simulink library "FF_Library"  (R2024b)
settings: Solver=VariableStepAuto  StartTime=0.0  StopTime=10.0  RelTol=1e-3
undefined symbols (not defined in the file or in its folder): Slope1, Slope2
libraries: simulink x60
(part 2 of 4)

== system FF_Library/Counter&Timer/CounterCycle_SourceZero ==
  Chart : Stateflow chart  TreatAsAtomicUnit=on
  Ts1 : Constant  Value=CounterCycle  OutDataTypeStr=Inherit: Inherit via back propagation  SampleTime=-1
      settings: AttributesFormatString=%<value>
      mask Display:
      | try
      | set_param(gcb,'AttributesFormatString','%<value>');% get the value name
      | % Constant=get_param(gcb,'Value');
      | % set_param(gcb,'Name',Constant,'ShowName','on');
      | end
      | try
      | Constant=get_param(gcb,'Value');
      | Constant_value=[Constant '.Value'];
      | Constant_type=[Constant '.DataType'];
      | Constant_value= evalin('base',Constant_value);% get the data name
      | Constant_type=evalin('base',Constant_type);% get the data type
      |           if strcmp(Constant_type,'boolean')||strcmp(Constant_type,'xpDT_Bool')% If the datatype is boolean
      |             if size(Constant_value)==[1 1]
      |                   if Constant_value==1
      |                     disp('True');
      |                   else
      |                     disp('False');
      |                   end
      |             else
      |                 disp(Constant_value);
      |             end
      |           else
      |              try
      |                  if mod(Constant_value,1)==0 &&(strcmp(Constant_type,'single')||strcmp(Constant_type,'xpDT_Single'))
      |                  fprintf('%.1f',Constant_value); %Display at least 1 decimal if DataType is 'single'
      |                  else
      |                  disp(Constant_value);
      |                  end
      |              catch
      |              disp(Constant_value);
      |              end
      |            end
      | catch
      |     try
      |        Constant_value= evalin('base',Constant);
      |        disp(num2str(Constant_value));
      |     catch
      |       color('blue');
      |       disp('NoData');
      |    end
      | end
      | %%  Created By Gmh 2018.06.28  %%
      | %%  Modified By Gmh 2018.10.24  %%
  Ts2 : Constant  Value=0  OutDataTypeStr=Inherit: Inherit via back propagation  SampleTime=-1
      settings: AttributesFormatString=%<value>
      mask Display:
      | try
      | set_param(gcb,'AttributesFormatString','%<value>');% get the value name
      | % Constant=get_param(gcb,'Value');
      | % set_param(gcb,'Name',Constant,'ShowName','on');
      | end
      | try
      | Constant=get_param(gcb,'Value');
      | Constant_value=[Constant '.Value'];
      | Constant_type=[Constant '.DataType'];
      | Constant_value= evalin('base',Constant_value);% get the data name
      | Constant_type=evalin('base',Constant_type);% get the data type
      |           if strcmp(Constant_type,'boolean')||strcmp(Constant_type,'xpDT_Bool')% If the datatype is boolean
      |             if size(Constant_value)==[1 1]
      |                   if Constant_value==1
      |                     disp('True');
      |                   else
      |                     disp('False');
      |                   end
      |             else
      |                 disp(Constant_value);
      |             end
      |           else
      |              try
      |                  if mod(Constant_value,1)==0 &&(strcmp(Constant_type,'single')||strcmp(Constant_type,'xpDT_Single'))
      |                  fprintf('%.1f',Constant_value); %Display at least 1 decimal if DataType is 'single'
      |                  else
      |                  disp(Constant_value);
      |                  end
      |              catch
      |              disp(Constant_value);
      |              end
      |            end
      | catch
      |     try
      |        Constant_value= evalin('base',Constant);
      |        disp(num2str(Constant_value));
      |     catch
      |       color('blue');
      |       disp('NoData');
      |    end
      | end
      | %%  Created By Gmh 2018.06.28  %%
      | %%  Modified By Gmh 2018.10.24  %%
  Ts3 : Constant  OutDataTypeStr=Inherit: Inherit via back propagation  SampleTime=-1
      settings: AttributesFormatString=%<value>
      mask Display:
      | try
      | set_param(gcb,'AttributesFormatString','%<value>');% get the value name
      | % Constant=get_param(gcb,'Value');
      | % set_param(gcb,'Name',Constant,'ShowName','on');
      | end
      | try
      | Constant=get_param(gcb,'Value');
      | Constant_value=[Constant '.Value'];
      | Constant_type=[Constant '.DataType'];
      | Constant_value= evalin('base',Constant_value);% get the data name
      | Constant_type=evalin('base',Constant_type);% get the data type
      |           if strcmp(Constant_type,'boolean')||strcmp(Constant_type,'xpDT_Bool')% If the datatype is boolean
      |             if size(Constant_value)==[1 1]
      |                   if Constant_value==1
      |                     disp('True');
      |                   else
      |                     disp('False');
      |                   end
      |             else
      |                 disp(Constant_value);
      |             end
      |           else
      |              try
      |                  if mod(Constant_value,1)==0 &&(strcmp(Constant_type,'single')||strcmp(Constant_type,'xpDT_Single'))
      |                  fprintf('%.1f',Constant_value); %Display at least 1 decimal if DataType is 'single'
      |                  else
      |                  disp(Constant_value);
      |                  end
      |              catch
      |              disp(Constant_value);
      |              end
      |            end
      | catch
      |     try
      |        Constant_value= evalin('base',Constant);
      |        disp(num2str(Constant_value));
      |     catch
      |       color('blue');
      |       disp('NoData');
      |    end
      | end
      | %%  Created By Gmh 2018.06.28  %%
      | %%  Modified By Gmh 2018.10.24  %%
  Cnt : Outport  VectorParamsAs1DForOutWhenUnconnected=off
  wires:
  Ts1/1 -> Chart/3(CounterCycle)
  Ts3/1 -> Chart/1(Enable)
  Ts2/1 -> Chart/2(InitValue)
  Chart/1(Cnt) -> Cnt/1

== system FF_Library/Counter&Timer/TIMER_RE ==
  note: y
  note: x1_out
  dT : Inport
  E : Inport  Port=2
  R : Inport  Port=3
  IV : Inport  Port=4
  x_in : Inport  Port=5
  Functionality : Subsystem
  y : Outport
  x_out : Outport  Port=2
  wires:
  dT/1 -> Functionality/4(dT)
  R/1 -> Functionality/2(R)
  Functionality/2(x_out) -> x_out/1
  IV/1 -> Functionality/3(IV)
  x_in/1 -> Functionality/5(x_in)
  Functionality/1(y) -> y/1
  E/1 -> Functionality/1(E)

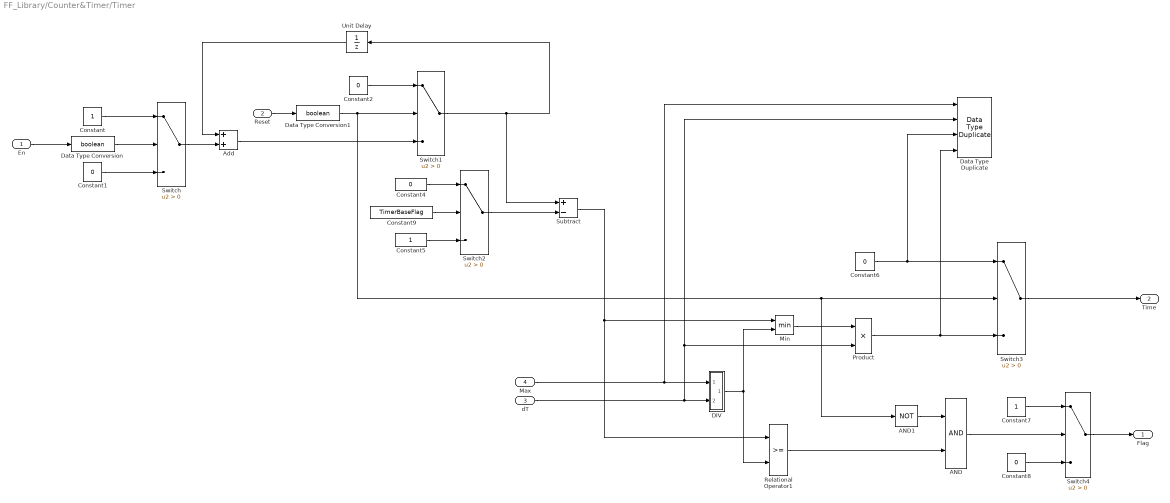
== system FF_Library/Counter&Timer/Timer ==
  En : Inport
  Reset : Inport  Port=2
  dT : Inport  Port=3
  Max : Inport  Port=4
  AND : Logic  AllPortsSameDT=off  OutDataTypeStr=boolean
  AND1 : Logic  Operator=NOT  AllPortsSameDT=off  OutDataTypeStr=boolean
  Add : Sum  OutDataTypeStr=single  SaturateOnIntegerOverflow=on
  Constant : Constant  OutDataTypeStr=boolean
  Constant{1..2,4,8} (4 alike) : Constant  Value=0  OutDataTypeStr=boolean
  Constant5 : Constant  OutDataTypeStr=boolean
  Constant6 : Constant  Value=0  OutDataTypeStr=Inherit: Inherit via back propagation
  Constant7 : Constant  OutDataTypeStr=boolean
  Constant9 : Constant  Value=TimerBaseFlag  OutDataTypeStr=boolean
  DIV : Subsystem  mask(DIV){MinRange=1e-15}
      mask prompts: MinRange "smallest allowed value to divide by"
      mask help:
      | 除法模块：
      | 带有除0保护。
      mask Display:
      | port_label('input',1,'×');
      | port_label('input',2,'÷');
      | port_label('output',1,'');
  Data Type Duplicate : DataTypeDuplicate  NumInputPorts=4
  Data Type Conversion : DataTypeConversion  OutDataTypeStr=boolean  RndMeth=Floor
  Data Type Conversion1 : DataTypeConversion  OutDataTypeStr=boolean  RndMeth=Floor
  Min : MinMax  Inputs=2
  Product : Product  OutDataTypeStr=Inherit: Inherit via back propagation  SaturateOnIntegerOverflow=on
  Relational Operator1 : RelationalOperator  OutDataTypeStr=boolean  RndMeth=Simplest  InputSameDT=off
  Subtract : Sum  Inputs=+-  SaturateOnIntegerOverflow=on
  Switch{,1..3} (4 alike) : Switch  Criteria=u2 > Threshold  InputSameDT=off
  Switch4 : Switch  Criteria=u2 > Threshold  OutDataTypeStr=boolean  InputSameDT=off
  Unit Delay : UnitDelay  InputProcessing=Columns as channels (frame based)  SampleTime=-1  HasFrameUpgradeWarning=on
  Flag : Outport
  Time : Outport  Port=2
  wires:
  Unit Delay/1 -> Add/1
  Constant9/1 -> Switch2/2
  Subtract/1 -> Relational Operator1/1, Min/1
  Add/1 -> Switch1/3
  Constant4/1 -> Switch2/1
  Switch3/1 -> Time/1
  DIV/1(Out1) -> Relational Operator1/2, Min/2
  Data Type Conversion1/1 -> Switch1/2, Switch3/2, AND1/1
  Constant2/1 -> Switch1/1
  Constant8/1 -> Switch4/3
  Constant6/1 -> Switch3/1, Data Type Duplicate/3
  Constant5/1 -> Switch2/3
  Constant/1 -> Switch/1
  AND1/1 -> AND/1
  Switch2/1 -> Subtract/2
  AND/1 -> Switch4/2
  Constant1/1 -> Switch/3
  Min/1 -> Product/1
  Constant7/1 -> Switch4/1
  Product/1 -> Switch3/3, Data Type Duplicate/4
  dT/1 -> Data Type Duplicate/2, Product/2, DIV/2(In2)
  Reset/1 -> Data Type Conversion1/1
  Switch1/1 -> Unit Delay/1, Subtract/1
  Switch/1 -> Add/2
  Data Type Conversion/1 -> Switch/2
  En/1 -> Data Type Conversion/1
  Switch4/1 -> Flag/1
  Max/1 -> Data Type Duplicate/1, DIV/1(In1)
  Relational Operator1/1 -> AND/2

== system FF_Library/Ctrl/INTEGRATORK_REL ==
  note: x_out
  note: B_max
  note: B_min
  note: y
  MX : Inport
  MN : Inport  Port=2
  K : Inport  Port=3
  dT : Inport  Port=4
  u : Inport  Port=5
  E : Inport  Port=6
  R : Inport  Port=7
  IV : Inport  Port=8
  x_in : Inport  Port=9
  Functionality : Subsystem
  y : Terminator
  B_min : Outport
  B_max : Outport  Port=2
  x_out : Outport  Port=3
  wires:
  Functionality/2(B_min) -> B_min/1
  Functionality/1(y) -> y/1
  u/1 -> Functionality/5(u)
  MX/1 -> Functionality/1(MX)
  E/1 -> Functionality/6(E)
  R/1 -> Functionality/7(R)
  MN/1 -> Functionality/2(MN)
  Functionality/3(B_max) -> B_max/1
  Functionality/4(x_out) -> x_out/1
  IV/1 -> Functionality/8(IV)
  K/1 -> Functionality/3(K)
  dT/1 -> Functionality/4(dT)
  x_in/1 -> Functionality/9(x_in)

== system FF_Library/Ctrl/INTEGRATORT_REL ==
  note: x_out
  note: B_max
  note: B_min
  note: y
  MX : Inport
  MN : Inport  Port=2
  T : Inport  Port=3
  dT : Inport  Port=4
  u : Inport  Port=5
  E : Inport  Port=6
  R : Inport  Port=7
  IV : Inport  Port=8
  x_in : Inport  Port=9
  Functionality : Subsystem
  y : Terminator
  B_min : Outport
  B_max : Outport  Port=2
  x_out : Outport  Port=3
  wires:
  Functionality/2(B_min) -> B_min/1
  Functionality/1(y) -> y/1
  u/1 -> Functionality/5(u)
  MX/1 -> Functionality/1(MX)
  E/1 -> Functionality/6(E)
  R/1 -> Functionality/7(R)
  MN/1 -> Functionality/2(MN)
  Functionality/3(B_max) -> B_max/1
  Functionality/4(x_out) -> x_out/1
  IV/1 -> Functionality/8(IV)
  T/1 -> Functionality/3(T)
  dT/1 -> Functionality/4(dT)
  x_in/1 -> Functionality/9(x_in)

== system FF_Library/Ctrl/Integrator ==
  Ini : Inport  OutDataTypeStr=boolean
  X : Inport  Port=2  OutDataTypeStr=single
  dT : Inport  Port=3  OutDataTypeStr=single
  Add1 : Sum
  Add2 : Sum
  Constant1 : Constant  Value=0  OutDataTypeStr=single
  Constant3 : Constant  Value=0  OutDataTypeStr=single
  Constant4 : Constant  Value=0.5  OutDataTypeStr=single
  Delay : Delay  DelayLength=1
  Delay1 : Delay  DelayLength=1
  Product : Product  Inputs=3
  Switch : Switch  Criteria=u2 > Threshold  OutDataTypeStr=single  SaturateOnIntegerOverflow=off  InputSameDT=off
  Switch1 : Switch  Criteria=u2 > Threshold  OutDataTypeStr=single  SaturateOnIntegerOverflow=off  InputSameDT=off
  Switch2 : Switch  Criteria=u2 > Threshold  OutDataTypeStr=single  SaturateOnIntegerOverflow=off  InputSameDT=off
  Y : Outport
  wires:
  dT/1 -> Product/1
  Delay/1 -> Switch1/3
  X/1 -> Delay/1, Switch/3
  Constant1/1 -> Switch2/1
  Constant3/1 -> Switch1/1, Switch/1
  Constant4/1 -> Product/2
  Add1/1 -> Y/1, Delay1/1
  Product/1 -> Add1/1
  Switch1/1 -> Add2/2
  Switch/1 -> Add2/1
  Add2/1 -> Product/3
  Delay1/1 -> Switch2/3
  Switch2/1 -> Add1/2
  Ini/1 -> Switch2/2, Switch1/2, Switch/2

== system FF_Library/Ctrl/PID ==
  err : Inport
  E : Inport  Port=2
  DefaultValue : Inport  Port=3
  FeedForward : Inport  Port=4
  Kp : Inport  Port=5
  Kd : Inport  Port=6
  Ki : Inport  Port=7
  Deadband : Inport  Port=8
  Ki_IV : Inport  Port=9
  UpperLimit : Inport  Port=10
  LowerLimit : Inport  Port=11
  Data Type Duplicate1 : DataTypeDuplicate  NumInputPorts=10
  PID : Subsystem
  PID_out : Outport
  wires:
  err/1 -> PID/1(err), Data Type Duplicate1/10
  Ki/1 -> PID/7(Ki), Data Type Duplicate1/5
  Deadband/1 -> PID/9(Deadband), Data Type Duplicate1/3
  Kp/1 -> PID/5(Kp), Data Type Duplicate1/7
  Kd/1 -> PID/6(Kd), Data Type Duplicate1/6
  FeedForward/1 -> PID/4(FeedForward), Data Type Duplicate1/8
  Ki_IV/1 -> PID/8(Ki_IV), Data Type Duplicate1/4
  PID/1(PID_out) -> PID_out/1
  E/1 -> PID/2(E)
  DefaultValue/1 -> PID/3(DefaultValue), Data Type Duplicate1/9
  LowerLimit/1 -> Data Type Duplicate1/1, PID/11(LowerLimit)
  UpperLimit/1 -> PID/10(UpperLimit), Data Type Duplicate1/2

== system FF_Library/Ctrl/PID_Norm ==
  Err : Inport
  Kp : Inport  Port=2
  Ki : Inport  Port=3
  Kd : Inport  Port=4
  Add : Sum  Inputs=+++  RndMeth=Nearest  SaturateOnIntegerOverflow=on
  Product : Product  RndMeth=Nearest  SaturateOnIntegerOverflow=on  OutDataTypeStr=Inherit: Same as first input
  Product1 : Product  RndMeth=Nearest  SaturateOnIntegerOverflow=on  OutDataTypeStr=Inherit: Same as first input
  Product2 : Product  RndMeth=Nearest  SaturateOnIntegerOverflow=on  OutDataTypeStr=Inherit: Same as first input
  Subtract : Sum  Inputs=+-  RndMeth=Nearest  SaturateOnIntegerOverflow=on  OutDataTypeStr=Inherit: Same as first input
  Subtract1 : Sum  RndMeth=Nearest  SaturateOnIntegerOverflow=on  OutDataTypeStr=Inherit: Same as first input
  Unit Delay : UnitDelay  SampleTime=-1  HasFrameUpgradeWarning=on
  Unit Delay1 : UnitDelay  SampleTime=-1  HasFrameUpgradeWarning=on
  PID_out : Outport
  wires:
  Product/1 -> Add/1
  Kp/1 -> Product/1
  Err/1 -> Subtract/1, Product2/1, Unit Delay/1, Product/2
  Subtract/1 -> Product1/1
  Product1/1 -> Add/2
  Ki/1 -> Product2/2
  Unit Delay/1 -> Subtract/2
  Product2/1 -> Subtract1/1
  Add/1 -> PID_out/1
  Kd/1 -> Product1/2
  Subtract1/1 -> Unit Delay1/1, Add/3
  Unit Delay1/1 -> Subtract1/2

== system FF_Library/Delay/TURNOFFDELAYSAMPLE ==
  note: x_out
  note: y
  n : Inport
  u : Inport  Port=2
  R : Inport  Port=3
  x_in : Inport  Port=4
  Functionality : Subsystem
  Rounding Function : Rounding  Operator=round
  y : Outport
  x_out : Outport  Port=2
  wires:
  x_in/1 -> Functionality/4(x_in)
  Functionality/2(x_out) -> x_out/1
  Functionality/1(y) -> y/1
  u/1 -> Functionality/2(u)
  n/1 -> Rounding Function/1
  R/1 -> Functionality/3(R)
  Rounding Function/1 -> Functionality/1(n)

== system FF_Library/Delay/TURNONDELAYSAMPLE ==
  note: x_out
  note: y
  R : Inport
  u : Inport  Port=2
  n : Inport  Port=3
  x_in : Inport  Port=4
  Functionality : Subsystem
  Rounding Function : Rounding  Operator=round
  y : Outport
  x_out : Outport  Port=2
  wires:
  x_in/1 -> Functionality/4(x_in)
  n/1 -> Rounding Function/1
  u/1 -> Functionality/2(u)
  R/1 -> Functionality/3(R)
  Functionality/2(x_out) -> x_out/1
  Functionality/1(y) -> y/1
  Rounding Function/1 -> Functionality/1(n)

== system FF_Library/Delay/TurnOffDeb ==
  u : Inport
  dT : Inport  Port=2
  T : Inport  Port=3
  AND : Logic  AllPortsSameDT=off  OutDataTypeStr=boolean
  AND1 : Logic  Operator=OR  AllPortsSameDT=off  OutDataTypeStr=boolean
  Constant : Constant  Value=0  OutDataTypeStr=Inherit: Inherit via back propagation
  Constant1 : Constant  Value=2  OutDataTypeStr=Inherit: Inherit via back propagation
  Constant2 : Constant  Value=0  OutDataTypeStr=Inherit: Inherit via back propagation
  DIV1 : Subsystem  mask(DIV){MinRange=1e-15}
      mask prompts: MinRange "smallest allowed value to divide by"
      mask help:
      | 除法模块：
      | 带有除0保护。
      mask Display:
      | port_label('input',1,'×');
      | port_label('input',2,'÷');
      | port_label('output',1,'');
  Data Type Duplicate : DataTypeDuplicate  NumInputPorts=4
  Max : MinMax  Function=max  Inputs=2
  NOT : Logic  Operator=NOT  AllPortsSameDT=off  OutDataTypeStr=boolean
  Relational Operator : RelationalOperator  Operator=>  OutDataTypeStr=boolean  RndMeth=Simplest  InputSameDT=off
  Subtract : Sum  Inputs=+-  SaturateOnIntegerOverflow=on
  Subtract2 : Sum  Inputs=+-  SaturateOnIntegerOverflow=on
  Switch : Switch  Criteria=u2 > Threshold  RndMeth=Nearest  InputSameDT=off
  Unit Delay : UnitDelay  SampleTime=-1  HasFrameUpgradeWarning=on
  Unit Delay1 : UnitDelay  SampleTime=-1  HasFrameUpgradeWarning=on
  y : Outport
  wires:
  u/1 -> Unit Delay/1, AND1/1, NOT/1
  NOT/1 -> AND/1
  Unit Delay/1 -> AND/2
  Relational Operator/1 -> AND1/2
  Constant/1 -> Relational Operator/2
  Switch/1 -> Data Type Duplicate/1, Unit Delay1/1, Relational Operator/1
  AND/1 -> Switch/2
  dT/1 -> DIV1/1(In1), Subtract/2, Data Type Duplicate/3
  Constant1/1 -> DIV1/2(In2), Data Type Duplicate/2
  T/1 -> Subtract2/1, Data Type Duplicate/4
  DIV1/1(Out1) -> Subtract2/2
  Unit Delay1/1 -> Subtract/1
  Constant2/1 -> Max/2
  Subtract/1 -> Max/1
  Max/1 -> Switch/3
  AND1/1 -> y/1
  Subtract2/1 -> Switch/1

== system FF_Library/Delay/TurnOffDelay ==
  X : Inport
  Delay : Inport  Port=2
  dT : Inport  Port=3
  Ini : Inport  Port=4
  ADD_blk1 : Sum  InputSameDT=on  OutDataTypeStr=Inherit: Same as first input
      settings: AttributesFormatString=Same input type: %<InputSameDT>
  AND : Logic  AllPortsSameDT=off  OutDataTypeStr=boolean
  CNST_FALSE : Constant  Value=0  OutDataTypeStr=boolean
  CNST_TRUE : Constant  OutDataTypeStr=boolean
  CNST_ZERO : Constant  Value=0  OutDataTypeStr=Inherit: Inherit via back propagation
  DLY_timer : UnitDelay  SampleTime=-1  HasFrameUpgradeWarning=on
      settings: AttributesFormatString=|
      | init = %<InitialCondition>
      | tsample = %<SampleTime>
  Delay1 : Delay  DelayLength=1  InputProcessing=Columns as channels (frame based)
  NOT1 : Logic  Operator=NOT  AllPortsSameDT=off  OutDataTypeStr=boolean
  OR : Logic  Operator=OR  AllPortsSameDT=off  OutDataTypeStr=boolean
  OR_blk : Logic  Operator=OR  OutDataTypeStr=boolean
  REL_blk : RelationalOperator  Operator=>  OutDataTypeStr=boolean  RndMeth=Simplest
  SWT_state : Switch  Criteria=u2 ~= 0  SaturateOnIntegerOverflow=off
      settings: AttributesFormatString=|
      | %<Criteria>
      | Same input type: %<InputSameDT>
  SWT_timer : Switch  Criteria=u2 ~= 0  SaturateOnIntegerOverflow=off
      settings: AttributesFormatString=|
      | %<Criteria>
      | Same input type: %<InputSameDT>
  Y : Outport  VectorParamsAs1DForOutWhenUnconnected=off
  wires:
  SWT_timer/1 -> REL_blk/1, DLY_timer/1
  Delay/1 -> REL_blk/2
  Ini/1 -> OR_blk/2
  X/1 -> OR/1, OR_blk/1
  DLY_timer/1 -> ADD_blk1/2
  OR_blk/1 -> SWT_timer/2
  ADD_blk1/1 -> SWT_timer/3
  dT/1 -> ADD_blk1/1
  CNST_ZERO/1 -> SWT_timer/1
  SWT_state/1 -> Delay1/1, Y/1
  CNST_FALSE/1 -> SWT_state/3
  CNST_TRUE/1 -> SWT_state/1
  REL_blk/1 -> NOT1/1
  OR/1 -> SWT_state/2
  AND/1 -> OR/2
  NOT1/1 -> AND/1
  Delay1/1 -> AND/2

== system FF_Library/Delay/TurnOnDeb ==
  u : Inport
  dT : Inport  Port=2
  T : Inport  Port=3
  AND : Logic  AllPortsSameDT=off  OutDataTypeStr=boolean
  AND1 : Logic  AllPortsSameDT=off  OutDataTypeStr=boolean
  Constant : Constant  Value=0  OutDataTypeStr=Inherit: Inherit via back propagation
  Constant1 : Constant  Value=2  OutDataTypeStr=Inherit: Inherit via back propagation
  Constant2 : Constant  Value=0  OutDataTypeStr=Inherit: Inherit via back propagation
  DIV : Subsystem  mask(DIV){MinRange=1e-15}
      mask prompts: MinRange "smallest allowed value to divide by"
      mask help:
      | 除法模块：
      | 带有除0保护。
      mask Display:
      | port_label('input',1,'×');
      | port_label('input',2,'÷');
      | port_label('output',1,'');
  Data Type Duplicate : DataTypeDuplicate  NumInputPorts=4
  Max : MinMax  Function=max  Inputs=2
  NOT1 : Logic  Operator=NOT  AllPortsSameDT=off  OutDataTypeStr=boolean
  Relational Operator : RelationalOperator  Operator=<=  OutDataTypeStr=boolean  RndMeth=Simplest  InputSameDT=off
  Subtract : Sum  Inputs=+-  SaturateOnIntegerOverflow=on
  Subtract1 : Sum  Inputs=+-  SaturateOnIntegerOverflow=on
  Switch : Switch  Criteria=u2 > Threshold  InputSameDT=off
  Unit Delay : UnitDelay  SampleTime=-1  HasFrameUpgradeWarning=on
  Unit Delay1 : UnitDelay  SampleTime=-1  HasFrameUpgradeWarning=on
  y : Outport
  wires:
  Constant2/1 -> Max/2
  Unit Delay1/1 -> Subtract1/1
  dT/1 -> DIV/1(In1), Subtract1/2, Data Type Duplicate/3
  Subtract1/1 -> Max/1
  AND1/1 -> y/1
  Switch/1 -> Data Type Duplicate/1, Unit Delay1/1, Relational Operator/1
  Unit Delay/1 -> NOT1/1
  T/1 -> Subtract/1, Data Type Duplicate/4
  Relational Operator/1 -> AND1/2
  DIV/1(Out1) -> Subtract/2
  AND/1 -> Switch/2
  Constant/1 -> Relational Operator/2
  u/1 -> AND/1, AND1/1, Unit Delay/1
  Max/1 -> Switch/3
  Constant1/1 -> DIV/2(In2), Data Type Duplicate/2
  Subtract/1 -> Switch/1
  NOT1/1 -> AND/2

== system FF_Library/Delay/TurnOnDelay ==
  X : Inport
  Delay : Inport  Port=2
  dT : Inport  Port=3
  Ini : Inport  Port=4
  ADD_blk1 : Sum  InputSameDT=on  OutDataTypeStr=Inherit: Same as first input
      settings: AttributesFormatString=Same input type: %<InputSameDT>
  CNST_FALSE : Constant  Value=0  OutDataTypeStr=boolean
  CNST_TRUE : Constant  OutDataTypeStr=boolean
  CNST_ZERO : Constant  Value=0  OutDataTypeStr=Inherit: Inherit via back propagation
  DLY_timer : UnitDelay  SampleTime=-1  HasFrameUpgradeWarning=on
      settings: AttributesFormatString=|
      | init = %<InitialCondition>
      | tsample = %<SampleTime>
  NOT_blk3 : Logic  Operator=NOT  OutDataTypeStr=boolean
  OR_blk : Logic  Operator=OR  OutDataTypeStr=boolean
  REL_blk : RelationalOperator  Operator=>  OutDataTypeStr=boolean  RndMeth=Simplest
  SWT_state : Switch  Criteria=u2 ~= 0  SaturateOnIntegerOverflow=off
      settings: AttributesFormatString=|
      | %<Criteria>
      | Same input type: %<InputSameDT>
  SWT_timer : Switch  Criteria=u2 ~= 0  SaturateOnIntegerOverflow=off
      settings: AttributesFormatString=|
      | %<Criteria>
      | Same input type: %<InputSameDT>
  Y : Outport  VectorParamsAs1DForOutWhenUnconnected=off
  wires:
  SWT_timer/1 -> REL_blk/1, DLY_timer/1
  Delay/1 -> REL_blk/2
  OR_blk/1 -> SWT_timer/2
  Ini/1 -> OR_blk/2
  NOT_blk3/1 -> OR_blk/1
  DLY_timer/1 -> ADD_blk1/2
  CNST_FALSE/1 -> SWT_state/3
  X/1 -> NOT_blk3/1
  ADD_blk1/1 -> SWT_timer/3
  CNST_TRUE/1 -> SWT_state/1
  dT/1 -> ADD_blk1/1
  CNST_ZERO/1 -> SWT_timer/1
  SWT_state/1 -> Y/1
  REL_blk/1 -> SWT_state/2

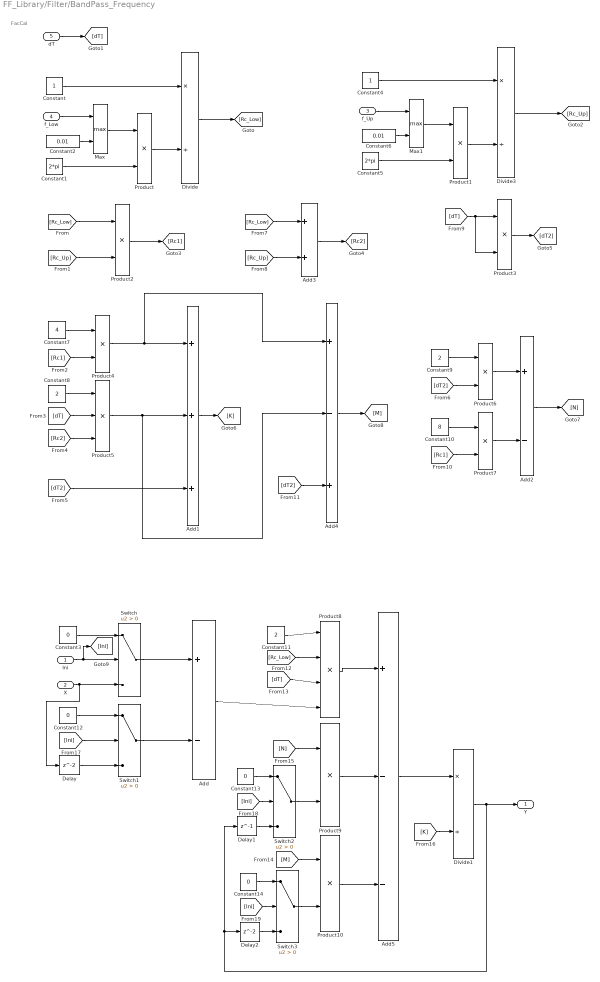
== system FF_Library/Filter/BandPass_Frequency ==
  note: FacCal
  Ini : Inport  OutDataTypeStr=boolean
  X : Inport  Port=2  OutDataTypeStr=single
  f_Up : Inport  Port=3  OutDataTypeStr=single
  f_Low : Inport  Port=4  OutDataTypeStr=single
  dT : Inport  Port=5  OutDataTypeStr=single
  Add : Sum  Inputs=+-
  Add1 : Sum  Inputs=+++
  Add2 : Sum  Inputs=+-
  Add3 : Sum
  Add4 : Sum  Inputs=+-+
  Add5 : Sum  Inputs=+--
  Constant : Constant  OutDataTypeStr=single
  Constant1 : Constant  Value=2*pi  OutDataTypeStr=single
  Constant10 : Constant  Value=8  OutDataTypeStr=single
  Constant11 : Constant  Value=2  OutDataTypeStr=single
  Constant{3,12..14} (4 alike) : Constant  Value=0  OutDataTypeStr=single
  Constant2 : Constant  Value=0.01  OutDataTypeStr=single
  Constant4 : Constant  OutDataTypeStr=single
  Constant5 : Constant  Value=2*pi  OutDataTypeStr=single
  Constant6 : Constant  Value=0.01  OutDataTypeStr=single
  Constant7 : Constant  Value=4  OutDataTypeStr=single
  Constant8 : Constant  Value=2  OutDataTypeStr=single
  Constant9 : Constant  Value=2  OutDataTypeStr=single
  Delay : Delay
  Delay1 : Delay  DelayLength=1
  Delay2 : Delay
  Divide : Product  Inputs=*/  OutDataTypeStr=single
  Divide1 : Product  Inputs=*/
  Divide3 : Product  Inputs=*/  OutDataTypeStr=single
  Max : MinMax  Function=max  Inputs=2
  Max1 : MinMax  Function=max  Inputs=2
  Product{,1..4,6..7,9..10} (9 alike) : Product
  Product5 : Product  Inputs=3
  Product8 : Product  Inputs=4
  Switch{,1..3} (4 alike) : Switch  Criteria=u2 > Threshold  OutDataTypeStr=single  SaturateOnIntegerOverflow=off  InputSameDT=off
  Y : Outport
  wires:
  [M] -> Product10/1
  Constant6/1 -> Max1/2
  [dT] -> Product5/2
  Product1/1 -> Divide3/2
  Add1/1 -> [K]
  [Ini] -> Switch1/2
  [dT] -> Product8/3
  Divide3/1 -> [Rc_Up]
  [dT2] -> Product6/2
  Product8/1 -> Add5/1
  Divide/1 -> [Rc_Low]
  Constant/1 -> Divide/1
  Switch1/1 -> Add/2
  Constant14/1 -> Switch3/1
  [dT2] -> Add1/3
  [Ini] -> Switch2/2
  Product2/1 -> [Rc1]
  Product9/1 -> Add5/2
  Constant9/1 -> Product6/1
  [dT] -> Product3/2, Product3/1
  Delay2/1 -> Switch3/3
  Constant2/1 -> Max/2
  Switch3/1 -> Product10/2
  Add3/1 -> [Rc2]
  [Ini] -> Switch3/2
  [Rc1] -> Product4/2
  Constant12/1 -> Switch1/1
  Product/1 -> Divide/2
  [Rc_Low] -> Add3/1
  Product7/1 -> Add2/2
  [K] -> Divide1/2
  Max/1 -> Product/1
  Product3/1 -> [dT2]
  Product6/1 -> Add2/1
  [dT2] -> Add4/3
  [Rc2] -> Product5/3
  Switch/1 -> Add/1
  Constant13/1 -> Switch2/1
  Constant10/1 -> Product7/1
  Add4/1 -> [M]
  dT/1 -> [dT]
  Delay1/1 -> Switch2/3
  f_Low/1 -> Max/1
  Product10/1 -> Add5/3
  Switch2/1 -> Product9/2
  [Rc_Up] -> Product2/2
  [Rc_Up] -> Add3/2
  Product5/1 -> Add4/2, Add1/2
  Add/1 -> Product8/4
  Constant3/1 -> Switch/1
  [Rc_Low] -> Product2/1
  Constant7/1 -> Product4/1
  [Rc_Low] -> Product8/2
  Max1/1 -> Product1/1
  Delay/1 -> Switch1/3
  [N] -> Product9/1
  Divide1/1 -> Y/1, Delay1/1, Delay2/1
  Constant11/1 -> Product8/1
  Product4/1 -> Add4/1, Add1/1
  Ini/1 -> [Ini], Switch/2
  Add2/1 -> [N]
  f_Up/1 -> Max1/1
  Constant4/1 -> Divide3/1
  Constant8/1 -> Product5/1
  Add5/1 -> Divide1/1
  [Rc1] -> Product7/2
  Constant5/1 -> Product1/2
  X/1 -> Switch/3, Delay/1
  Constant1/1 -> Product/2

== system FF_Library/Filter/DIGITALLOWPASS_RE ==
  note: y
  note: x_out
  m : Inport
  u : Inport  Port=2
  E : Inport  Port=3
  R : Inport  Port=4
  IV : Inport  Port=5
  x_in : Inport  Port=6
  Functionality : Subsystem  Description=FLP
  x : Terminator
  y : Outport
  x_out : Outport  Port=2
  wires:
  IV/1 -> Functionality/5(IV)
  E/1 -> Functionality/3(E)
  Functionality/2(x_out) -> x/1, x_out/1
  Functionality/1(y) -> y/1
  R/1 -> Functionality/4(R)
  u/1 -> Functionality/2(u)
  m/1 -> Functionality/1(m)
  x_in/1 -> Functionality/6(x_in)

== system FF_Library/Filter/HIGHPASST_RE ==
  note: x1_out
  note: y
  note: x2_out
  T : Inport
  TD : Inport  Port=2
  dT : Inport  Port=3
  u : Inport  Port=4
  E : Inport  Port=5
  R : Inport  Port=6
  IV : Inport  Port=7
  x1_in : Inport  Port=8
  x2_in : Inport  Port=9
  Functionality : Subsystem  Description=FLP
  y : Outport
  x1_out : Outport  Port=2
  x2_out : Outport  Port=3
  wires:
  E/1 -> Functionality/5(E)
  Functionality/3(x2_out) -> x2_out/1
  T/1 -> Functionality/1(T)
  R/1 -> Functionality/6(R)
  x2_in/1 -> Functionality/9(x2_in)
  TD/1 -> Functionality/2(TD)
  dT/1 -> Functionality/3(dT)
  u/1 -> Functionality/4(u)
  Functionality/2(x1_out) -> x1_out/1
  IV/1 -> Functionality/7(IV)
  x1_in/1 -> Functionality/8(x1_in)
  Functionality/1(y) -> y/1

== system FF_Library/Filter/LOWPASSK_RE ==
  note: x_out
  note: y
  K : Inport
  dT : Inport  Port=2
  u : Inport  Port=3
  E : Inport  Port=4
  R : Inport  Port=5
  IV : Inport  Port=6
  x_in : Inport  Port=7
  Divide : Product  Inputs=**
  Functionality : Subsystem  Description=FLP
      settings: PostSaveFcn=;
  check_mrange : Subsystem
  m_calc_SS : SignalSpecification  OutDataTypeStr=double
  x : Terminator
  y : Outport
  x_out : Outport  Port=2
  wires:
  Functionality/1(y) -> y/1
  Functionality/2(x_out) -> x_out/1, x/1
  u/1 -> Functionality/2(u)
  E/1 -> Functionality/3(E)
  R/1 -> Functionality/4(R)
  IV/1 -> Functionality/5(IV)
  x_in/1 -> Functionality/6(x_in)
  K/1 -> Divide/1
  dT/1 -> Divide/2
  Divide/1 -> check_mrange/1(m), m_calc_SS/1
  m_calc_SS/1 -> Functionality/1(m)

== system FF_Library/Filter/LOWPASSSECORD_RE ==
  note: x2_out
  note: x1_out
  note: y
  T : Inport
  D : Inport  Port=2
  dT : Inport  Port=3
  u : Inport  Port=4
  E : Inport  Port=5
  R : Inport  Port=6
  IV1 : Inport  Port=7
  IV2 : Inport  Port=8
  x1_in : Inport  Port=9
  x2_in : Inport  Port=10
  Functionality : Subsystem
  x1 : Terminator
  x2 : Terminator
  y : Outport
  x1_out : Outport  Port=2
  x2_out : Outport  Port=3
  wires:
  x2_in/1 -> Functionality/10(x2_in)
  x1_in/1 -> Functionality/9(x1_in)
  Functionality/1(y) -> y/1
  Functionality/2(x1_out) -> x1_out/1, x1/1
  Functionality/3(x2_out) -> x2_out/1, x2/1
  T/1 -> Functionality/1(T)
  D/1 -> Functionality/2(D)
  dT/1 -> Functionality/3(dT)
  u/1 -> Functionality/4(u)
  E/1 -> Functionality/5(E)
  R/1 -> Functionality/6(R)
  IV1/1 -> Functionality/7(IV1)
  IV2/1 -> Functionality/8(IV2)

== system FF_Library/Filter/LOWPASST_RE ==
  note: x_out
  note: y
  T : Inport
  dT : Inport  Port=2
  u : Inport  Port=3
  E : Inport  Port=4
  R : Inport  Port=5
  IV : Inport  Port=6
  x_in : Inport  Port=7
  Divide : Product  Inputs=*/
  Functionality : Subsystem  Description=FLP
      settings: PostSaveFcn=;
  check_mrange : Subsystem
  m_calc_SS : SignalSpecification  OutDataTypeStr=double
  x : Terminator
  y : Outport
  x_out : Outport  Port=2
  wires:
  Functionality/1(y) -> y/1
  Functionality/2(x_out) -> x_out/1, x/1
  u/1 -> Functionality/2(u)
  E/1 -> Functionality/3(E)
  R/1 -> Functionality/4(R)
  IV/1 -> Functionality/5(IV)
  x_in/1 -> Functionality/6(x_in)
  dT/1 -> Divide/1
  Divide/1 -> check_mrange/1(m), m_calc_SS/1
  m_calc_SS/1 -> Functionality/1(m)
  T/1 -> Divide/2

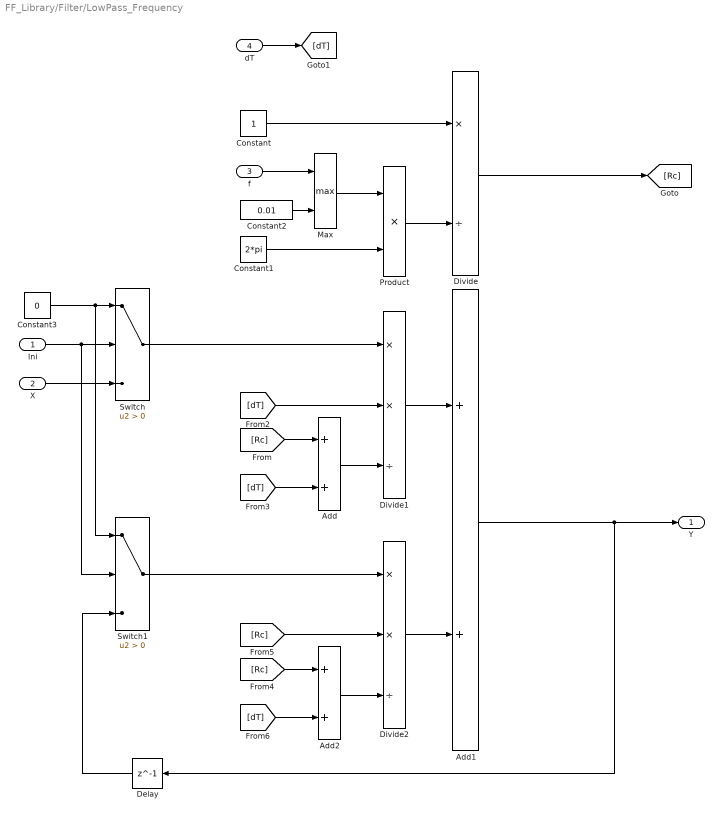
== system FF_Library/Filter/LowPass_Frequency ==
  Ini : Inport  OutDataTypeStr=boolean
  X : Inport  Port=2  OutDataTypeStr=single
  f : Inport  Port=3  OutDataTypeStr=single
  dT : Inport  Port=4  OutDataTypeStr=single
  Add : Sum
  Add1 : Sum  OutDataTypeStr=single
  Add2 : Sum
  Constant : Constant  OutDataTypeStr=single
  Constant1 : Constant  Value=2*pi  OutDataTypeStr=single
  Constant2 : Constant  Value=0.01  OutDataTypeStr=single
  Constant3 : Constant  Value=0  OutDataTypeStr=single
  Delay : Delay  DelayLength=1
  Divide : Product  Inputs=*/  OutDataTypeStr=single
  Divide1 : Product  Inputs=**/  OutDataTypeStr=single
  Divide2 : Product  Inputs=**/  OutDataTypeStr=single
  Max : MinMax  Function=max  Inputs=2
  Product : Product
  Switch : Switch  Criteria=u2 > Threshold  OutDataTypeStr=single  SaturateOnIntegerOverflow=off  InputSameDT=off
  Switch1 : Switch  Criteria=u2 > Threshold  OutDataTypeStr=single  SaturateOnIntegerOverflow=off  InputSameDT=off
  Y : Outport
  wires:
  [dT] -> Add/2
  Divide2/1 -> Add1/2
  [dT] -> Divide1/2
  X/1 -> Switch/3
  [dT] -> Add2/2
  Max/1 -> Product/1
  Product/1 -> Divide/2
  [Rc] -> Divide2/2
  Divide1/1 -> Add1/1
  Add/1 -> Divide1/3
  Divide/1 -> [Rc]
  Constant1/1 -> Product/2
  Switch/1 -> Divide1/1
  Constant/1 -> Divide/1
  [Rc] -> Add/1
  Ini/1 -> Switch/2, Switch1/2
  Constant3/1 -> Switch/1, Switch1/1
  f/1 -> Max/1
  Delay/1 -> Switch1/3
  [Rc] -> Add2/1
  Add2/1 -> Divide2/3
  Add1/1 -> Delay/1, Y/1
  Constant2/1 -> Max/2
  dT/1 -> [dT]
  Switch1/1 -> Divide2/1

== system FF_Library/Filter/LowPass_K ==
  Ini : Inport  OutDataTypeStr=boolean
  X : Inport  Port=2  OutDataTypeStr=single
  K : Inport  Port=3  OutDataTypeStr=single
  dT : Inport  Port=4  OutDataTypeStr=single
  Add : Sum  Inputs=+-
  Add1 : Sum  OutDataTypeStr=single
  Constant : Constant  OutDataTypeStr=single
  Constant3 : Constant  Value=0  OutDataTypeStr=single
  Delay : Delay  DelayLength=1
  Divide1 : Product  Inputs=**  OutDataTypeStr=single
  Divide2 : Product  Inputs=**  OutDataTypeStr=single
  Divide3 : Product  Inputs=**  OutDataTypeStr=single
  Switch : Switch  Criteria=u2 > Threshold  OutDataTypeStr=single  SaturateOnIntegerOverflow=off  InputSameDT=off
  Switch1 : Switch  Criteria=u2 > Threshold  OutDataTypeStr=single  SaturateOnIntegerOverflow=off  InputSameDT=off
  Y : Outport
  wires:
  Switch/1 -> Divide1/1
  Constant/1 -> Add/1
  Divide3/1 -> Add/2, Divide1/2
  Constant3/1 -> Switch1/1, Switch/1
  Delay/1 -> Switch1/3
  Ini/1 -> Switch1/2, Switch/2
  Add/1 -> Divide2/2
  K/1 -> Divide3/2
  Add1/1 -> Y/1, Delay/1
  X/1 -> Switch/3
  dT/1 -> Divide3/1
  Switch1/1 -> Divide2/1
  Divide2/1 -> Add1/2
  Divide1/1 -> Add1/1

== system FF_Library/Filter/Moving_Average ==
  u : Inport
  Reset : Inport  Port=2
  InitialValue : Inport  Port=3
  Moving Average : Stateflow chart  TreatAsAtomicUnit=on
  y : Outport
  wires:
  Moving Average/1(average) -> y/1
  u/1 -> Moving Average/1(u)
  Reset/1 -> Moving Average/2(Reset)
  InitialValue/1 -> Moving Average/3(InitialValue)

== system FF_Library/Filter/T-Filter ==
  Tup : Inport
  Tdown : Inport  Port=2
  u : Inport  Port=3
  dT : Inport  Port=4
  Add : Sum  SaturateOnIntegerOverflow=on
  Constant1 : Constant  Value=0  OutDataTypeStr=Inherit: Inherit via back propagation
  DIV1 : Subsystem  mask(DIV){MinRange=1e-15}
      mask prompts: MinRange "smallest allowed value to divide by"
      mask help:
      | 除法模块：
      | 带有除0保护。
      mask Display:
      | port_label('input',1,'×');
      | port_label('input',2,'÷');
      | port_label('output',1,'');
  Data Type Duplicate : DataTypeDuplicate  NumInputPorts=3
  Data Type Duplicate1 : DataTypeDuplicate  NumInputPorts=3
  Data Type Conversion : DataTypeConversion  OutDataTypeStr=single  RndMeth=Floor
  Data Type Conversion1 : DataTypeConversion  OutDataTypeStr=single  RndMeth=Floor
  Data Type Conversion2 : DataTypeConversion  RndMeth=Floor
  Delay : Delay  DelayLength=1  InitialConditionSource=Input port
      settings: InputPortMap=u0,p4
  InitValue : Constant  Value=0  OutDataTypeStr=Inherit: Inherit via back propagation
  Max : MinMax  Function=max  Inputs=2
  Product : Product  SaturateOnIntegerOverflow=on
  Relational Operator : RelationalOperator  OutDataTypeStr=boolean  RndMeth=Simplest  InputSameDT=off
  Subtract1 : Sum  Inputs=+-  SaturateOnIntegerOverflow=on
  Switch : Switch  Criteria=u2 > Threshold  InputSameDT=off
  Switch1 : Switch  Criteria=u2 > Threshold  InputSameDT=off
  bChooseInitValue : Constant  Value=0  OutDataTypeStr=boolean
  y : Outport
  wires:
  u/1 -> Data Type Duplicate1/2, Data Type Conversion/1
  Data Type Conversion/1 -> Subtract1/1, Switch/3
  dT/1 -> Data Type Duplicate/3, Product/2, Max/1
  Subtract1/1 -> Product/1, Relational Operator/1
  Product/1 -> DIV1/1(In1)
  Max/1 -> DIV1/2(In2)
  Switch1/1 -> Max/2
  DIV1/1(Out1) -> Add/1
  Constant1/1 -> Relational Operator/2
  Relational Operator/1 -> Switch1/2
  Tup/1 -> Data Type Duplicate/2, Switch1/1
  Tdown/1 -> Data Type Duplicate/1, Switch1/3
  bChooseInitValue/1 -> Switch/2
  InitValue/1 -> Data Type Duplicate1/1, Data Type Conversion1/1
  Data Type Conversion1/1 -> Switch/1
  Add/1 -> Delay/1, Data Type Conversion2/1
  Data Type Conversion2/1 -> y/1, Data Type Duplicate1/3
  Delay/1 -> Add/2, Subtract1/2
  Switch/1 -> Delay/2

== system FF_Library/Limit/ACCUMULATOR_REL ==
  note: x_out
  note: B_max
  note: B_min
  note: y
  MX : Inport
  MN : Inport  Port=2
  u : Inport  Port=3
  E : Inport  Port=4
  R : Inport  Port=5
  IV : Inport  Port=6
  x_in : Inport  Port=7
  Functionality : Subsystem
  y : Terminator
  B_min : Outport
  B_max : Outport  Port=2
  x_out : Outport  Port=3
  wires:
  IV/1 -> Functionality/6(IV)
  Functionality/4(x_out) -> x_out/1
  Functionality/3(B_max) -> B_max/1
  MN/1 -> Functionality/2(MN)
  R/1 -> Functionality/5(R)
  E/1 -> Functionality/4(E)
  MX/1 -> Functionality/1(MX)
  u/1 -> Functionality/3(u)
  Functionality/1(y) -> y/1
  Functionality/2(B_min) -> B_min/1
  x_in/1 -> Functionality/7(x_in)

== system FF_Library/Limit/DIFFERENCELIMITER ==
  LU : Inport
  LD : Inport  Port=2
  u : Inport  Port=3
  E : Inport  Port=4
  R : Inport  Port=5
  IV : Inport  Port=6
  x_in : Inport  Port=7
  Functionality : Subsystem  mask(Functionality_DIFFERENCELIMITER_SIMULINK){}
  y : Terminator
  B_min : Outport
  B_max : Outport  Port=2
  x_out : Outport  Port=3
  wires:
  E/1 -> Functionality/3(E)
  Functionality/2(B_min) -> B_min/1
  Functionality/1(y) -> y/1
  IV/1 -> Functionality/5(IV)
  x_in/1 -> Functionality/6(x_in)
  LU/1 -> Functionality/1(LU)
  Functionality/4(x_out) -> x_out/1
  R/1 -> Functionality/4(R)
  u/1 -> Functionality/7(u)
  Functionality/3(B_max) -> B_max/1
  LD/1 -> Functionality/2(LD)

== system FF_Library/Limit/DeadBan_RE ==
  UMAX : Inport
  UMIN : Inport  Port=2
  u : Inport  Port=3
  Data Type Duplicate : DataTypeDuplicate
  Functionality : Subsystem
  Signal Conversion : SignalConversion  ConversionOutput=Contiguous copy  OverrideOpt=off
  y : Outport
  wires:
  Signal Conversion/1 -> y/1
  u/1 -> Data Type Duplicate/2, Functionality/3(u)
  UMIN/1 -> Functionality/2(UMIN)
  Functionality/1(y) -> Signal Conversion/1, Data Type Duplicate/1
  UMAX/1 -> Functionality/1(UMAX)

== system FF_Library/Limit/DeadBand ==
  R : Inport
  L : Inport  Port=2
  u : Inport  Port=3
  Add1 : Sum  Inputs=-+  InputSameDT=on  SaturateOnIntegerOverflow=on
  Subsystem : Subsystem
  Switch1 : Switch  Criteria=u2 > Threshold  InputSameDT=off
  Unit Delay : UnitDelay  SampleTime=-1  HasFrameUpgradeWarning=on
      settings: AttributesFormatString=%<InitialCondition>
  y : Outport
  wires:
  R/1 -> Subsystem/1(MX)
  Unit Delay/1 -> Add1/1, Switch1/1
  Subsystem/1(y) -> Switch1/2
  u/1 -> Switch1/3, Add1/2
  L/1 -> Subsystem/2(MN)
  Switch1/1 -> y/1, Unit Delay/1
  Add1/1 -> Subsystem/3(u)

== system FF_Library/Limit/GRADIENTLIMITER ==
  LU : Inport
  LD : Inport  Port=2
  dT : Inport  Port=3
  u : Inport  Port=4
  E : Inport  Port=5
  R : Inport  Port=6
  IV : Inport  Port=7
  x_in : Inport  Port=8
  Functionality : Subsystem
  y : Terminator
  B_min : Outport
  B_max : Outport  Port=2
  x_out : Outport  Port=3
  wires:
  LD/1 -> Functionality/2(LD)
  E/1 -> Functionality/5(E)
  Functionality/2(B_min) -> B_min/1
  Functionality/3(B_max) -> B_max/1
  x_in/1 -> Functionality/8(x_in)
  LU/1 -> Functionality/1(LU)
  dT/1 -> Functionality/3(dT)
  R/1 -> Functionality/6(R)
  IV/1 -> Functionality/7(IV)
  Functionality/4(x_out) -> x_out/1
  Functionality/1(y) -> y/1
  u/1 -> Functionality/4(u)

== system FF_Library/Limit/Hysteresis ==
  LSP : Inport
  RSP : Inport  Port=2
  U : Inport  Port=3
  R : Inport  Port=4
  RV : Inport  Port=5
  0 : UnitDelay  SampleTime=-1  HasFrameUpgradeWarning=on
  NOT : Logic  Operator=OR  AllPortsSameDT=off  OutDataTypeStr=boolean
  Relational Operator1 : RelationalOperator  Operator=>  OutDataTypeStr=boolean  RndMeth=Simplest
  Relational Operator2 : RelationalOperator  Operator=<  OutDataTypeStr=boolean  RndMeth=Simplest
  Switch : Switch  Criteria=u2 > Threshold  InputSameDT=off
  Switch1 : Switch  Criteria=u2 > Threshold  InputSameDT=off
  y : Outport
  wires:
  U/1 -> Relational Operator2/1, Relational Operator1/1
  RSP/1 -> Relational Operator1/2
  LSP/1 -> Relational Operator2/2
  Relational Operator2/1 -> NOT/1
  Relational Operator1/1 -> Switch/1, NOT/2
  NOT/1 -> Switch/2
  RV/1 -> Switch1/1
  R/1 -> Switch1/2
  Switch1/1 -> Switch/3
  0/1 -> Switch1/3
  Switch/1 -> y/1, 0/1

== system FF_Library/Limit/Hysteresis_Left ==
  X : Inport  OutDataTypeStr=single
  Thd : Inport  Port=2  OutDataTypeStr=single
  HysDwn : Inport  Port=3  OutDataTypeStr=single
  AND : Logic  AllPortsSameDT=off  OutDataTypeStr=boolean
  Delay : Delay  DelayLength=1  InputProcessing=Columns as channels (frame based)
  OR_blk : Logic  Operator=OR  OutDataTypeStr=boolean
  REL_blk : RelationalOperator  OutDataTypeStr=boolean  RndMeth=Simplest
  REL_blk1 : RelationalOperator  OutDataTypeStr=boolean  RndMeth=Simplest
  SUB_blk : Sum  InputSameDT=on  OutDataTypeStr=Inherit: Same as first input
      settings: AttributesFormatString=Same input type: %<InputSameDT>
  Y : Outport  OutDataTypeStr=boolean  VectorParamsAs1DForOutWhenUnconnected=off
  wires:
  SUB_blk/1 -> REL_blk1/2
  [Thd] -> REL_blk/2
  Delay/1 -> AND/2
  AND/1 -> OR_blk/2
  REL_blk/1 -> AND/1
  HysDwn/1 -> SUB_blk/2
  Thd/1 -> [Thd], SUB_blk/1
  X/1 -> REL_blk1/1, REL_blk/1
  REL_blk1/1 -> OR_blk/1
  OR_blk/1 -> Delay/1, Y/1

== system FF_Library/Limit/Hysteresis_Right ==
  X : Inport  OutDataTypeStr=single
  Thd : Inport  Port=2  OutDataTypeStr=single
  HysDwn : Inport  Port=3  OutDataTypeStr=single
  AND : Logic  AllPortsSameDT=off  OutDataTypeStr=boolean
  Delay : Delay  DelayLength=1  InputProcessing=Columns as channels (frame based)
  OR_blk : Logic  Operator=OR  OutDataTypeStr=boolean
  REL_blk : RelationalOperator  OutDataTypeStr=boolean  RndMeth=Simplest
  REL_blk1 : RelationalOperator  OutDataTypeStr=boolean  RndMeth=Simplest
  SUB_blk : Sum  Inputs=+-  InputSameDT=on  OutDataTypeStr=Inherit: Same as first input
      settings: AttributesFormatString=Same input type: %<InputSameDT>
  Y : Outport  OutDataTypeStr=boolean  VectorParamsAs1DForOutWhenUnconnected=off
  wires:
  SUB_blk/1 -> REL_blk/2
  X/1 -> REL_blk1/1, REL_blk/1
  REL_blk/1 -> AND/1
  HysDwn/1 -> SUB_blk/2
  Thd/1 -> [Thd], SUB_blk/1
  AND/1 -> OR_blk/2
  Delay/1 -> AND/2
  REL_blk1/1 -> OR_blk/1
  [Thd] -> REL_blk1/2
  OR_blk/1 -> Delay/1, Y/1

== system FF_Library/Limit/Limit ==
  MX : Inport
  MN : Inport  Port=2
  u : Inport  Port=3
  AND : Logic  AllPortsSameDT=off  OutDataTypeStr=boolean
  Data Type Conversion : DataTypeConversion  RndMeth=Floor
  Max : MinMax  Function=max  Inputs=2  InputSameDT=on
  Min : MinMax  Inputs=2  InputSameDT=on
  NOT : Logic  Operator=NOT  AllPortsSameDT=off  OutDataTypeStr=boolean
  Relational Operator : RelationalOperator  Operator=>  OutDataTypeStr=boolean  RndMeth=Simplest
  Relational Operator1 : RelationalOperator  Operator=<  OutDataTypeStr=boolean  RndMeth=Simplest
  y : Outport
  B_max : Outport  Port=2
  B_min : Outport  Port=3
  wires:
  MX/1 -> Relational Operator/2, Min/1
  Max/1 -> Min/2
  u/1 -> Relational Operator1/1, Relational Operator/1, Max/1
  MN/1 -> Relational Operator1/2, Max/2
  Relational Operator/1 -> B_max/1, NOT/1
  Relational Operator1/1 -> AND/2
  NOT/1 -> AND/1
  AND/1 -> B_min/1
  Min/1 -> Data Type Conversion/1
  Data Type Conversion/1 -> y/1

== system FF_Library/Limit/Ramp ==
  u : Inport
  RisingRamp : Inport  Port=2
  FailingRamp : Inport  Port=3
  dT : Inport  Port=4
  BaseValue : Inport  Port=5
  Abs : Abs  RndMeth=Nearest
  Abs1 : Abs  RndMeth=Nearest
  Add : Sum  RndMeth=Nearest  SaturateOnIntegerOverflow=on
  Add1 : Sum  Inputs=+-  RndMeth=Nearest  SaturateOnIntegerOverflow=on  OutDataTypeStr=Inherit: Same as first input
  Constant : Constant  Value=-1  OutDataTypeStr=single
      settings: AttributesFormatString=%<OutDataTypeStr>
      settings: MoveFcn=|
      | try
      | ConstantValue = get_param(gcb,'Value');
      | if isempty(str2num(ConstantValue))
      | set_param(gcb,'name',ConstantValue);
      | end
      | end
  Data Type Duplicate : DataTypeDuplicate
  Data Type Conversion : DataTypeConversion  RndMeth=Nearest
      settings: AttributesFormatString=%<OutDataTypeStr>
  MinMax : MinMax  Inputs=2  RndMeth=Nearest  SaturateOnIntegerOverflow=on
  MinMax1 : MinMax  Function=max  Inputs=2  OutDataTypeStr=Inherit: Inherit via back propagation  RndMeth=Nearest  SaturateOnIntegerOverflow=on
  Product : Product  RndMeth=Nearest  SaturateOnIntegerOverflow=on  OutDataTypeStr=Inherit: Same as first input
  Product1 : Product  RndMeth=Nearest  SaturateOnIntegerOverflow=on  OutDataTypeStr=Inherit: Same as first input
  Product2 : Product  OutDataTypeStr=Inherit: Inherit via back propagation  RndMeth=Nearest  SaturateOnIntegerOverflow=on
  y : Outport
  wires:
  MinMax1/1 -> Add/1
  Add/1 -> Data Type Conversion/1
  u/1 -> Add1/1, Data Type Duplicate/2
  dT/1 -> Product/2, Product1/1
  BaseValue/1 -> Add1/2, Add/2
  Add1/1 -> MinMax/2
  Product2/1 -> MinMax1/1
  Abs1/1 -> Product1/2
  Constant/1 -> Product2/2
  Abs/1 -> Product/1
  Product1/1 -> MinMax/1
  Product/1 -> Product2/1
  Data Type Conversion/1 -> Data Type Duplicate/1, y/1
  MinMax/1 -> MinMax1/2
  FailingRamp/1 -> Abs/1
  RisingRamp/1 -> Abs1/1

== system FF_Library/Memory/BooleanHold ==
  u : Inport
  Count : Subsystem
  Logical Operator : Logic  Operator=OR  AllPortsSameDT=off  OutDataTypeStr=boolean
  Logical Operator5 : Logic  AllPortsSameDT=off  OutDataTypeStr=boolean
  Relational Operator1 : RelationalOperator  Operator=~=  OutDataTypeStr=boolean  RndMeth=Simplest
  Unit_Delay1 : UnitDelay  SampleTime=-1  HasFrameUpgradeWarning=on
      settings: AttributesFormatString=init=%<X0>
  y : Outport
  wires:
  Count/2(FALSE_debounce) -> Logical Operator5/1
  Unit_Delay1/1 -> Logical Operator5/2, Relational Operator1/2
  Logical Operator/1 -> y/1, Unit_Delay1/1
  Relational Operator1/1 -> Count/2(Edge)
  u/1 -> Relational Operator1/1, Count/1(u)
  Count/1(TRUE_debounce) -> Logical Operator/1
  Logical Operator5/1 -> Logical Operator/2

== system FF_Library/Memory/DELTAONESTEP ==
  u : Inport
  R : Inport  Port=2
  IV : Inport  Port=3
  x_in : Inport  Port=4
  Functionality : Subsystem
  fcg : simulink/Ports & Subsystems/Function-Call Generator  sample_time=-1  numberOfIterations=1  DisallowWideOutput=off
  y : Outport
  x_out : Outport  Port=2
  wires:
  fcg/1 -> Functionality/Trigger
  x_in/1 -> Functionality/4(x_in)
  IV/1 -> Functionality/3(IV)
  R/1 -> Functionality/2(R)
  u/1 -> Functionality/1(u)
  Functionality/2(x_out) -> x_out/1
  Functionality/1(y) -> y/1

== system FF_Library/Memory/DIFFERENCEQUOTIENT ==
  note: x_out
  note: y
  dT : Inport
  u : Inport  Port=2
  R : Inport  Port=3
  IV : Inport  Port=4
  x_in : Inport  Port=5
  Functionality : Subsystem
  fcg : simulink/Ports & Subsystems/Function-Call Generator  sample_time=-1  numberOfIterations=1  DisallowWideOutput=off
  x : Terminator
  y : Outport
  x_out : Outport  Port=2
  wires:
  fcg/1 -> Functionality/Trigger
  Functionality/2(x_out) -> x/1, x_out/1
  dT/1 -> Functionality/1(dT)
  u/1 -> Functionality/2(u)
  R/1 -> Functionality/3(R)
  IV/1 -> Functionality/4(IV)
  Functionality/1(y) -> y/1
  x_in/1 -> Functionality/5(x_in)

== system FF_Library/Memory/EDGEBI ==
  u : Inport  OutDataTypeStr=boolean
  Relational Operator1 : RelationalOperator  Operator=~=  OutDataTypeStr=boolean  RndMeth=Simplest
  Unit Delay : UnitDelay  SampleTime=-1  HasFrameUpgradeWarning=on
  y : Outport  OutDataTypeStr=boolean
  wires:
  Relational Operator1/1 -> y/1
  u/1 -> Unit Delay/1, Relational Operator1/1
  Unit Delay/1 -> Relational Operator1/2

== system FF_Library/Memory/EDGEFALLING ==
  u : Inport  OutDataTypeStr=boolean
  Logical Operator : Logic  AllPortsSameDT=off  OutDataTypeStr=boolean
  Logical Operator1 : Logic  Operator=NOT  AllPortsSameDT=off  OutDataTypeStr=boolean
  Unit_Delay : UnitDelay  SampleTime=-1  HasFrameUpgradeWarning=on
      settings: AttributesFormatString=init=%<X0>
  y : Outport  OutDataTypeStr=boolean
  wires:
  Unit_Delay/1 -> Logical Operator/2
  u/1 -> Unit_Delay/1, Logical Operator1/1
  Logical Operator1/1 -> Logical Operator/1
  Logical Operator/1 -> y/1

== system FF_Library/Memory/EDGERAISING ==
  u : Inport  OutDataTypeStr=boolean
  Logical Operator : Logic  AllPortsSameDT=off  OutDataTypeStr=boolean
  Logical Operator1 : Logic  Operator=NOT  AllPortsSameDT=off  OutDataTypeStr=boolean
  Unit_Delay1 : UnitDelay  SampleTime=-1  HasFrameUpgradeWarning=on
      settings: AttributesFormatString=init=%<X0>
  y : Outport  OutDataTypeStr=boolean
  wires:
  Logical Operator/1 -> y/1
  Logical Operator1/1 -> Logical Operator/1
  u/1 -> Unit_Delay1/1, Logical Operator/2
  Unit_Delay1/1 -> Logical Operator1/1

== system FF_Library/Memory/LoopHold ==
  u : Inport
  Init : Inport  Port=2
  Add : Sum  SaturateOnIntegerOverflow=on
  Constant : Constant  Value=0  OutDataTypeStr=Inherit: Inherit via back propagation  SampleTime=-1
  Constant1 : Constant  Value=0  OutDataTypeStr=Inherit: Inherit via back propagation  SampleTime=-1
  Constant2 : Constant  OutDataTypeStr=Inherit: Inherit via back propagation  SampleTime=-1
  Constant3 : Constant  Value=LoopHold  OutDataTypeStr=uint16
  Delay : Delay  DelayLength=1  InitialCondition=0
  Delay1 : Delay  DelayLength=1  InitialConditionSource=Input port  InitialCondition=0
      settings: InputPortMap=u0,p4
  Detect Change : simulink/Logic and Bit Operations/Detect Change  vinit=0  OutDataTypeStr=boolean
  Relational Operator : RelationalOperator  OutDataTypeStr=boolean  RndMeth=Simplest  InputSameDT=off
  Saturation Dynamic : simulink/Discontinuities/Saturation Dynamic  OutMin=[]  OutMax=[]  OutDataTypeStr=Inherit: Same as second input  OutDataType=fixdt(1, 16)  OutScaling=2^-10  DoSatur=off
  Switch : Switch  Criteria=u2 > Threshold  InputSameDT=off
  Switch1 : Switch  Criteria=u2 > Threshold  InputSameDT=off
  y : Outport
  wires:
  Add/1 -> Saturation Dynamic/2
  Init/1 -> Delay1/2
  [LoopHold] -> Relational Operator/2
  Delay1/1 -> Switch1/3
  Constant1/1 -> Switch/1
  Saturation Dynamic/1 -> Switch/3
  Detect Change/1 -> Switch/2
  Constant/1 -> Saturation Dynamic/3
  Delay/1 -> Add/2
  Constant2/1 -> Add/1
  Constant3/1 -> Saturation Dynamic/1, [LoopHold]
  Relational Operator/1 -> Switch1/2
  Switch/1 -> Relational Operator/1, Delay/1
  u/1 -> Switch1/1, Detect Change/1
  Switch1/1 -> y/1, Delay1/1
